simulink model "test"  (R2022a)
settings: Solver=VariableStepAuto  StartTime=0.0  StopTime=1000  RelTol=1e-3
settings Model: Creator=anthony  LastModifiedBy=anthony

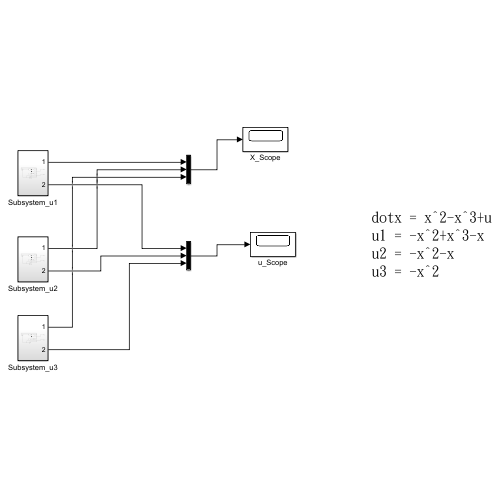
[thumbnail: Simulink's stored preview of the top-level diagram]
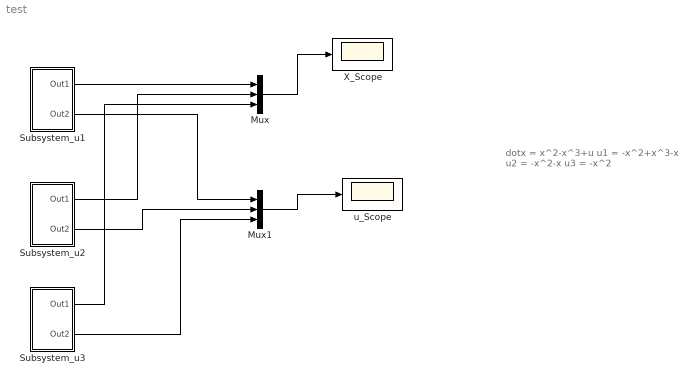
== system test ==
  note: dotx = x^2-x^3+u
      | u1 = -x^2+x^3-x
      | u2 = -x^2-x
      | u3 = -x^2
  Mux : Mux  Inputs=3
  Mux1 : Mux  Inputs=3
  Subsystem_u1 : Subsystem
  Subsystem_u2 : Subsystem
  Subsystem_u3 : Subsystem
  X_Scope : Scope
  u_Scope : Scope
  wires:
  Mux/1 -> X_Scope/1
  Mux1/1 -> u_Scope/1
  Subsystem_u1/1(Out1) -> Mux/1
  Subsystem_u1/2(Out2) -> Mux1/1
  Subsystem_u2/1(Out1) -> Mux/2
  Subsystem_u2/2(Out2) -> Mux1/2
  Subsystem_u3/1(Out1) -> Mux/3
  Subsystem_u3/2(Out2) -> Mux1/3

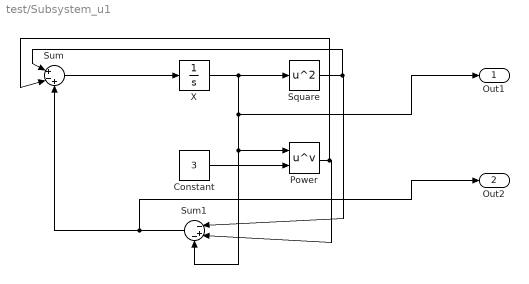
== system test/Subsystem_u1 ==
  Constant : Constant  Value=3
  Power : Math  Operator=pow
  Square : Math  Operator=square
  Sum : Sum  Inputs=|+-+
  Sum1 : Sum  Inputs=|-+-
  X : Integrator  InitialCondition=10
  Out1 : Outport
  Out2 : Outport  Port=2
  wires:
  Sum/1 -> X/1
  Square/1 -> Sum/1, Sum1/1
  Constant/1 -> Power/2
  Sum1/1 -> Out2/1, Sum/3
  Power/1 -> Sum/2, Sum1/2
  X/1 -> Out1/1, Sum1/3, Power/1, Square/1

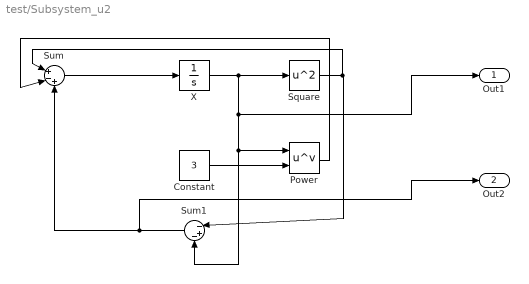
== system test/Subsystem_u2 ==
  Constant : Constant  Value=3
  Power : Math  Operator=pow
  Square : Math  Operator=square
  Sum : Sum  Inputs=|+-+
  Sum1 : Sum  Inputs=|-+-
  X : Integrator  InitialCondition=10
  Out1 : Outport
  Out2 : Outport  Port=2
  wires:
  X/1 -> Square/1, Power/1, Sum1/3, Out1/1
  Power/1 -> Sum/2
  Sum1/1 -> Sum/3, Out2/1
  Constant/1 -> Power/2
  Square/1 -> Sum1/1, Sum/1
  Sum/1 -> X/1

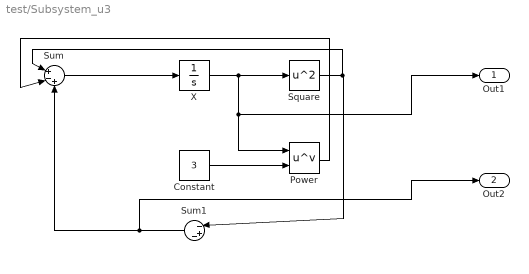
== system test/Subsystem_u3 ==
  Constant : Constant  Value=3
  Power : Math  Operator=pow
  Square : Math  Operator=square
  Sum : Sum  Inputs=|+-+
  Sum1 : Sum  Inputs=|-+-
  X : Integrator  InitialCondition=10
  Out1 : Outport
  Out2 : Outport  Port=2
  wires:
  Sum/1 -> X/1
  Square/1 -> Sum/1, Sum1/1
  Constant/1 -> Power/2
  Sum1/1 -> Out2/1, Sum/3
  Power/1 -> Sum/2
  X/1 -> Out1/1, Power/1, Square/1
